simulink model "position_pid"  (R2019a)
settings: Solver=VariableStepAuto  StartTime=0.0  StopTime=200  RelTol=1e-3
undefined symbols (not defined in the file or in its folder): Ki
settings Model: Creator=intel  LastModifiedBy=intel

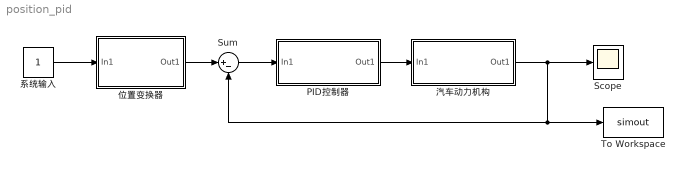
== system position_pid ==
  PID控制器 : Subsystem
  Scope : Scope
  Sum : Sum  Inputs=|+-
  To Workspace : ToWorkspace  VariableName=simout  SaveFormat=Timeseries  SampleTime=-1
  位置变换器 : Subsystem
  汽车动力机构 : Subsystem
  系统输入 : Constant
  wires:
  系统输入/1 -> 位置变换器/1(In1)
  PID控制器/1(Out1) -> 汽车动力机构/1(In1)
  位置变换器/1(Out1) -> Sum/1
  Sum/1 -> PID控制器/1(In1)
  汽车动力机构/1(Out1) -> Scope/1, To Workspace/1, Sum/2

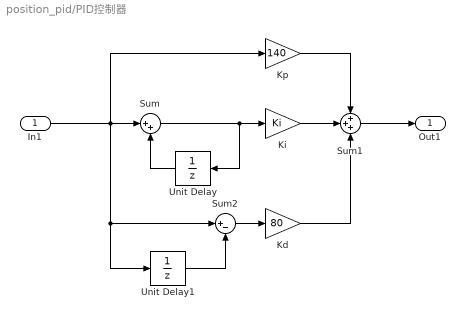
== system position_pid/PID控制器 ==
  In1 : Inport
  Kd : Gain  Gain=80
  Ki : Gain  Gain=Ki
  Kp : Gain  Gain=140
  Sum : Sum  Inputs=|++
  Sum1 : Sum  Inputs=+++
  Sum2 : Sum  Inputs=|+-
  Unit Delay : UnitDelay  SampleTime=0.02  HasFrameUpgradeWarning=on
  Unit Delay1 : UnitDelay  SampleTime=0.02  HasFrameUpgradeWarning=on
  Out1 : Outport
  wires:
  In1/1 -> Unit Delay1/1, Sum2/1, Kp/1, Sum/1
  Sum/1 -> Ki/1, Unit Delay/1
  Unit Delay/1 -> Sum/2
  Ki/1 -> Sum1/2
  Kp/1 -> Sum1/1
  Unit Delay1/1 -> Sum2/2
  Sum2/1 -> Kd/1
  Kd/1 -> Sum1/3
  Sum1/1 -> Out1/1

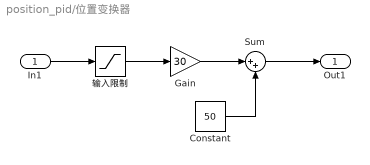
== system position_pid/位置变换器 ==
  In1 : Inport
  Constant : Constant  Value=50
  Gain : Gain  Gain=30
  Sum : Sum  Inputs=|++
  输入限制 : Saturate  UpperLimit=1  LowerLimit=0
  Out1 : Outport
  wires:
  In1/1 -> 输入限制/1
  输入限制/1 -> Gain/1
  Gain/1 -> Sum/1
  Sum/1 -> Out1/1
  Constant/1 -> Sum/2

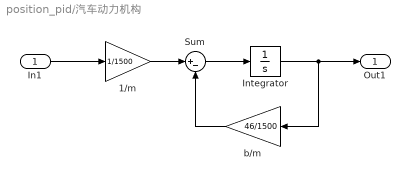
== system position_pid/汽车动力机构 ==
  In1 : Inport
  1/m : Gain  Gain=1/1500
  Integrator : Integrator
  Sum : Sum  Inputs=|+-
  b/m : Gain  Gain=46/1500
  Out1 : Outport
  wires:
  In1/1 -> 1/m/1
  1/m/1 -> Sum/1
  Sum/1 -> Integrator/1
  b/m/1 -> Sum/2
  Integrator/1 -> b/m/1, Out1/1
